simulink model "simulink_a1"  (R2020a)
settings: Solver=FixedStepAuto  StartTime=0.0  StopTime=10.0  FixedStep=1e-3  RelTol=1e-3  EnableMultiTasking=on
undefined symbols (not defined in the file): D0, D1, D10, D11, D12, D13, D2, D3, D4, D5, D6, D7, D8, D9, PTA0, PTA1, PTA2, PTB23, PTB9, PTC16, PTC17, PTC2, PTC3, PTC4, PTD0, PTD1, PTD2, PTD3
libraries: frdmk64flib x18
settings Model: ExtModeTrigDuration=5  Creator=eotte  LastModifiedBy=eotte
settings OptimizationCC: EnhancedBackFolding=on  PassReuseOutputArgsAs=Individual arguments  ZeroExternalMemoryAtStartup=off  ZeroInternalMemoryAtStartup=off  MaxStackSize=64  OptimizeBlockOrder=speed  DifferentSizesBufferReuse=on  OptimizationCustomize=off  EfficientTunableParamExpr=on
settings DebuggingCC: ParameterTunabilityLossMsg=error
settings HardwareCC: ProdBitPerPointer=32  ProdBitPerSizeT=32  ProdBitPerPtrDiffT=32  ProdLargestAtomicInteger=Long  ProdLargestAtomicFloat=Double  ProdWordSize=32  ProdHWDeviceType=ARM Compatible->ARM Cortex
settings SFSimCC: MATLABDynamicMemAlloc=off
settings RTWCC: SystemTargetFile=ert.tlc  HardwareBoard=NXP FRDM-K64F  TemplateMakefile=ert_default_tmf  Toolchain=GNU Tools for ARM Embedded Processors
settings CodeAppCC: ForceParamTrailComments=on  IgnoreCustomStorageClasses=off  OperatorAnnotations=on  SimulinkDataObjDesc=on  SFDataObjDesc=on  InsertBlockDesc=on

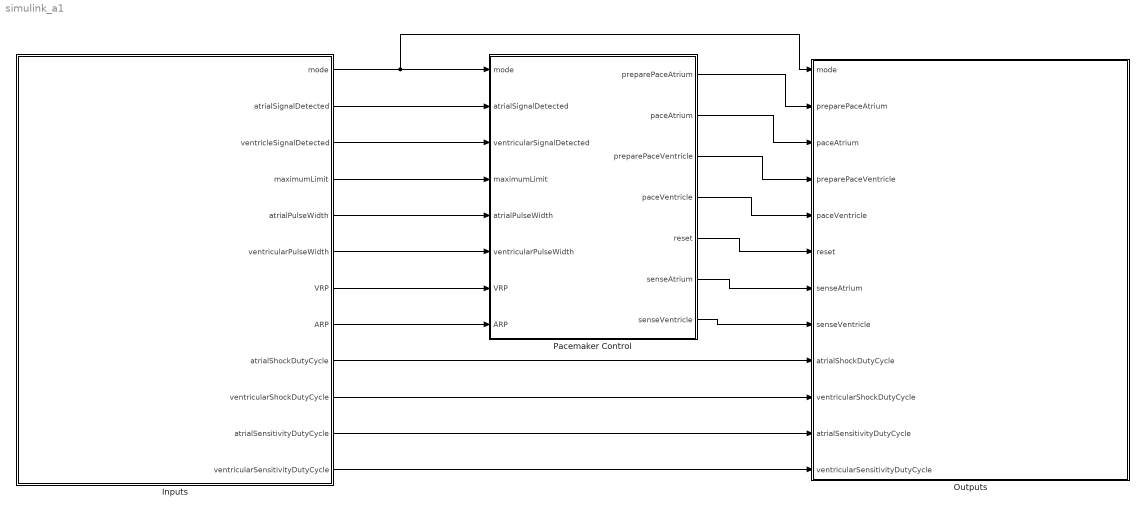
== system simulink_a1 ==
  Inputs : Subsystem
  Outputs : Subsystem
  Pacemaker Control : Stateflow chart  TreatAsAtomicUnit=on
  wires:
  Pacemaker Control/1(preparePaceAtrium) -> Outputs/2(preparePaceAtrium)
  Pacemaker Control/3(preparePaceVentricle) -> Outputs/4(preparePaceVentricle)
  Pacemaker Control/2(paceAtrium) -> Outputs/3(paceAtrium)
  Pacemaker Control/4(paceVentricle) -> Outputs/5(paceVentricle)
  Inputs/1(mode) -> Pacemaker Control/1(mode), Outputs/1(mode)
  Pacemaker Control/5(reset) -> Outputs/6(reset)
  Inputs/2(atrialSignalDetected) -> Pacemaker Control/2(atrialSignalDetected)
  Inputs/3(ventricleSignalDetected) -> Pacemaker Control/3(ventricularSignalDetected)
  Inputs/12(ventricularSensitivityDutyCycle) -> Outputs/12(ventricularSensitivityDutyCycle)
  Inputs/11(atrialSensitivityDutyCycle) -> Outputs/11(atrialSensitivityDutyCycle)
  Inputs/10(ventricularShockDutyCycle) -> Outputs/10(ventricularShockDutyCycle)
  Inputs/9(atrialShockDutyCycle) -> Outputs/9(atrialShockDutyCycle)
  Inputs/4(maximumLimit) -> Pacemaker Control/4(maximumLimit)
  Inputs/5(atrialPulseWidth) -> Pacemaker Control/5(atrialPulseWidth)
  Inputs/6(ventricularPulseWidth) -> Pacemaker Control/6(ventricularPulseWidth)
  Inputs/7(VRP) -> Pacemaker Control/7(VRP)
  Inputs/8(ARP) -> Pacemaker Control/8(ARP)
  Pacemaker Control/6(senseAtrium) -> Outputs/7(senseAtrium)
  Pacemaker Control/7(senseVentricle) -> Outputs/8(senseVentricle)

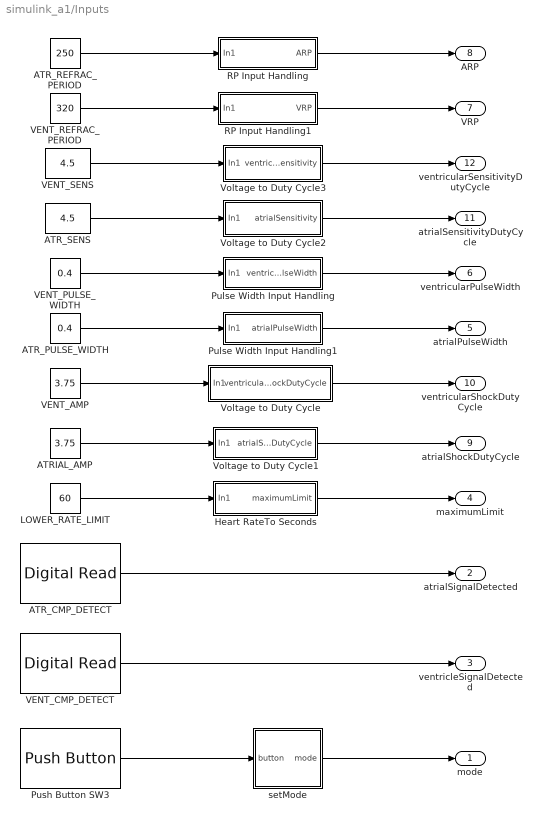
== system simulink_a1/Inputs ==
  ATRIAL_AMP : Constant  Value=3.75
  ATR_CMP_DETECT : frdmk64flib/Digital Read  Whichpin=PTC16 (D0)  SampleTime=-1
  ATR_PULSE_WIDTH : Constant  Value=0.4
  ATR_REFRAC_PERIOD : Constant  Value=250
  ATR_SENS : Constant  Value=4.5
  Heart RateTo Seconds : Subsystem
  LOWER_RATE_LIMIT : Constant  Value=60
  Pulse Width Input Handling : Subsystem
  Pulse Width Input Handling1 : Subsystem
  Push Button SW3 : frdmk64flib/Push Button  Whichswitch=SW3  SampleTime1=-1
  RP Input Handling : Subsystem
  RP Input Handling1 : Subsystem
  VENT_AMP : Constant  Value=3.75
  VENT_CMP_DETECT : frdmk64flib/Digital Read  Whichpin=PTC17 (D1)  SampleTime=-1
  VENT_PULSE_WIDTH : Constant  Value=0.4
  VENT_REFRAC_PERIOD : Constant  Value=320
  VENT_SENS : Constant  Value=4.5
  Voltage to Duty Cycle : Subsystem
  Voltage to Duty Cycle1 : Subsystem
  Voltage to Duty Cycle2 : Subsystem
  Voltage to Duty Cycle3 : Subsystem
  setMode : Stateflow chart  TreatAsAtomicUnit=on
  mode : Outport
  atrialSignalDetected : Outport  Port=2
  ventricleSignalDetected : Outport  Port=3
  maximumLimit : Outport  Port=4
  atrialPulseWidth : Outport  Port=5
  ventricularPulseWidth : Outport  Port=6
  VRP : Outport  Port=7
  ARP : Outport  Port=8
  atrialShockDutyCycle : Outport  Port=9
  ventricularShockDutyCycle : Outport  Port=10
  atrialSensitivityDutyCycle : Outport  Port=11
  ventricularSensitivityDutyCycle : Outport  Port=12
  wires:
  setMode/1(mode) -> mode/1
  Push Button SW3/1 -> setMode/1(button)
  ATR_CMP_DETECT/1 -> atrialSignalDetected/1
  VENT_CMP_DETECT/1 -> ventricleSignalDetected/1
  ATRIAL_AMP/1 -> Voltage to Duty Cycle1/1(In1)
  VENT_AMP/1 -> Voltage to Duty Cycle/1(In1)
  VENT_SENS/1 -> Voltage to Duty Cycle3/1(In1)
  ATR_SENS/1 -> Voltage to Duty Cycle2/1(In1)
  VENT_PULSE_WIDTH/1 -> Pulse Width Input Handling/1(In1)
  LOWER_RATE_LIMIT/1 -> Heart RateTo Seconds/1(In1)
  Heart RateTo Seconds/1(maximumLimit) -> maximumLimit/1
  Voltage to Duty Cycle/1(ventricularShockDutyCycle) -> ventricularShockDutyCycle/1
  Voltage to Duty Cycle1/1(atrialShockDutyCycle) -> atrialShockDutyCycle/1
  Voltage to Duty Cycle3/1(ventricularSensitivity) -> ventricularSensitivityDutyCycle/1
  Voltage to Duty Cycle2/1(atrialSensitivity) -> atrialSensitivityDutyCycle/1
  Pulse Width Input Handling/1(ventricularPulseWidth) -> ventricularPulseWidth/1
  Pulse Width Input Handling1/1(atrialPulseWidth) -> atrialPulseWidth/1
  ATR_PULSE_WIDTH/1 -> Pulse Width Input Handling1/1(In1)
  RP Input Handling1/1(VRP) -> VRP/1
  RP Input Handling/1(ARP) -> ARP/1
  ATR_REFRAC_PERIOD/1 -> RP Input Handling/1(In1)
  VENT_REFRAC_PERIOD/1 -> RP Input Handling1/1(In1)

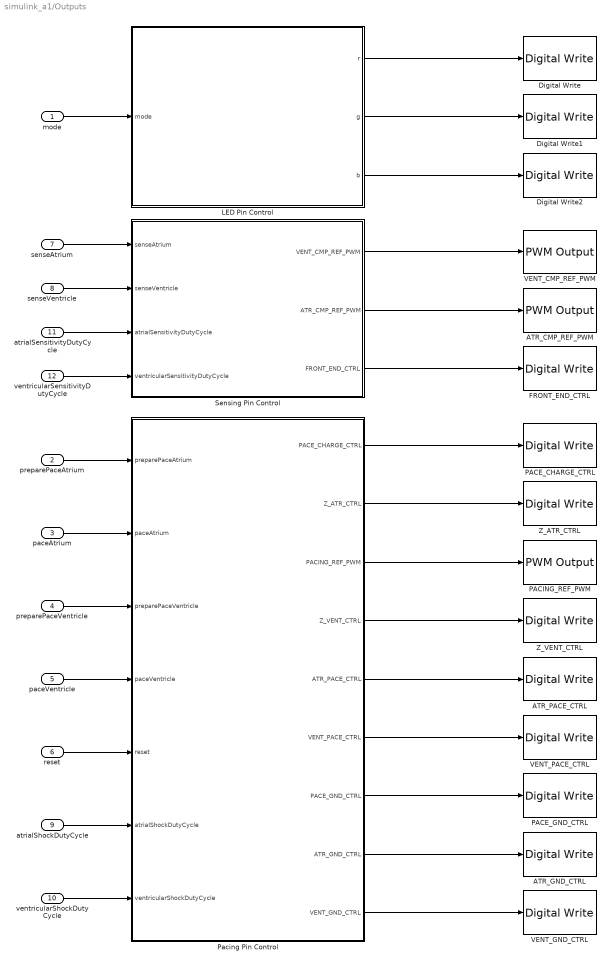
== system simulink_a1/Outputs ==
  mode : Inport
  preparePaceAtrium : Inport  Port=2
  paceAtrium : Inport  Port=3
  preparePaceVentricle : Inport  Port=4
  paceVentricle : Inport  Port=5
  reset : Inport  Port=6
  senseAtrium : Inport  Port=7
  senseVentricle : Inport  Port=8
  atrialShockDutyCycle : Inport  Port=9
  ventricularShockDutyCycle : Inport  Port=10
  atrialSensitivityDutyCycle : Inport  Port=11
  ventricularSensitivityDutyCycle : Inport  Port=12
  ATR_CMP_REF_PWM : frdmk64flib/PWM Output  Whichpin=PTC2 (D6)  InitialFrequency=2000  InitialDutyCycle=0
  ATR_GND_CTRL : frdmk64flib/Digital Write  Whichpin=PTD2 (D11)
  ATR_PACE_CTRL : frdmk64flib/Digital Write  Whichpin=PTA0 (D8)
  Digital Write : frdmk64flib/Digital Write  Whichpin=RED_LED
  Digital Write1 : frdmk64flib/Digital Write  Whichpin=GREEN_LED
  Digital Write2 : frdmk64flib/Digital Write  Whichpin=BLUE_LED
  FRONT_END_CTRL : frdmk64flib/Digital Write  Whichpin=PTD1 (D13)
  LED Pin Control : Stateflow chart  TreatAsAtomicUnit=on
  PACE_CHARGE_CTRL : frdmk64flib/Digital Write  Whichpin=PTB9 (D2)
  PACE_GND_CTRL : frdmk64flib/Digital Write  Whichpin=PTD0 (D10)
  PACING_REF_PWM : frdmk64flib/PWM Output  Whichpin=PTA2 (D5)  InitialFrequency=2000  InitialDutyCycle=0
  Pacing Pin Control : Stateflow chart  TreatAsAtomicUnit=on
      settings: PortSchema="{\"entries\":[{\"content\":{\"sides\":[{\"content\":{\"connectorIds\":[\"In1\",\"In2\",\"In3\",\"In4\",\"In5\",\"In6\",\"In7\"]},\"type\":\"ConnectorPlacement.EquallySpacedRectSide\",\"uuid\":\"92253962-87e9-4e7c-bcdb-24e58fe0c055\"},{\"content\":{\"connectorIds\":[\"Out2\",\"Out8\",\"Out5\",\"Out9\",\"Out3\",\"Out7\",\"Out4\",\"Out1\",\"Out6\"],\"side\":\"RIGHT\"},\"type\":\"ConnectorPlacement.EquallySpacedRectSide\",\"uuid\":\"4cb9541d-32ff-4bb4-8e4b-d9f1d7e76c76\"},{\"content\":{\"connectorIds\":[],\"side\":\"TOP\"},\"type\":\"ConnectorPlacement.EquallySpacedRectSide\",\"uuid\":\"cc690cb9-25b8-4ee8-ae3f-a22909f5e3a8\"},{\"content\":{\"connectorIds\":[],\"side\":\"BOTTOM\"},\"type\":\"ConnectorPlacement.EquallySpacedRectSide\",\"uuid\":\"0aa6c860-c953-4b2e-baf5-040a508b9d07\"}]},\"type\":\"ConnectorPlacement.EquallySpacedConnector\",\"uuid\":\"d7c6b2d5-ade3-439b-b1ea-d68e76d328ac\"}],\"packageUris\":[\"http://schema.mathworks.com/mf0/Connector/19700101\"],\"version\":\"1.0\"}"
  Sensing Pin Control : Stateflow chart  TreatAsAtomicUnit=on
      settings: PortSchema="{\"entries\":[{\"content\":{\"sides\":[{\"content\":{\"connectorIds\":[\"In1\",\"In2\",\"In3\",\"In4\"]},\"type\":\"ConnectorPlacement.EquallySpacedRectSide\",\"uuid\":\"f0f6a072-4109-4fa4-bc82-6d6350130513\"},{\"content\":{\"connectorIds\":[\"Out3\",\"Out2\",\"Out1\"],\"side\":\"RIGHT\"},\"type\":\"ConnectorPlacement.EquallySpacedRectSide\",\"uuid\":\"04a191da-9ef7-404f-bbc7-e2275fa0f798\"},{\"content\":{\"connectorIds\":[],\"side\":\"TOP\"},\"type\":\"ConnectorPlacement.EquallySpacedRectSide\",\"uuid\":\"3258143e-ec04-4818-a8fd-7397dd93120a\"}]},\"type\":\"ConnectorPlacement.EquallySpacedConnector\",\"uuid\":\"abd9187b-7230-471c-b20b-6fa4748c984d\"}],\"packageUris\":[\"http://schema.mathworks.com/mf0/Connector/19700101\"],\"version\":\"1.0\"}"
  VENT_CMP_REF_PWM : frdmk64flib/PWM Output  Whichpin=PTA1 (D3)  InitialFrequency=2000  InitialDutyCycle=0
  VENT_GND_CTRL : frdmk64flib/Digital Write  Whichpin=PTD3 (D12)
  VENT_PACE_CTRL : frdmk64flib/Digital Write  Whichpin=PTC4 (D9)
  Z_ATR_CTRL : frdmk64flib/Digital Write  Whichpin=PTB23 (D4)
  Z_VENT_CTRL : frdmk64flib/Digital Write  Whichpin=PTC3 (D7)
  wires:
  preparePaceAtrium/1 -> Pacing Pin Control/1(preparePaceAtrium)
  paceAtrium/1 -> Pacing Pin Control/2(paceAtrium)
  preparePaceVentricle/1 -> Pacing Pin Control/3(preparePaceVentricle)
  paceVentricle/1 -> Pacing Pin Control/4(paceVentricle)
  Pacing Pin Control/1(ATR_GND_CTRL) -> ATR_GND_CTRL/1
  Pacing Pin Control/2(PACE_CHARGE_CTRL) -> PACE_CHARGE_CTRL/1
  Pacing Pin Control/3(ATR_PACE_CTRL) -> ATR_PACE_CTRL/1
  Pacing Pin Control/5(PACING_REF_PWM) -> PACING_REF_PWM/1
  Pacing Pin Control/8(Z_ATR_CTRL) -> Z_ATR_CTRL/1
  Pacing Pin Control/4(PACE_GND_CTRL) -> PACE_GND_CTRL/1
  Pacing Pin Control/6(VENT_GND_CTRL) -> VENT_GND_CTRL/1
  Pacing Pin Control/9(Z_VENT_CTRL) -> Z_VENT_CTRL/1
  Pacing Pin Control/7(VENT_PACE_CTRL) -> VENT_PACE_CTRL/1
  reset/1 -> Pacing Pin Control/5(reset)
  atrialShockDutyCycle/1 -> Pacing Pin Control/6(atrialShockDutyCycle)
  ventricularShockDutyCycle/1 -> Pacing Pin Control/7(ventricularShockDutyCycle)
  LED Pin Control/2(g) -> Digital Write1/1
  LED Pin Control/1(r) -> Digital Write/1
  LED Pin Control/3(b) -> Digital Write2/1
  mode/1 -> LED Pin Control/1(mode)
  senseVentricle/1 -> Sensing Pin Control/2(senseVentricle)
  senseAtrium/1 -> Sensing Pin Control/1(senseAtrium)
  atrialSensitivityDutyCycle/1 -> Sensing Pin Control/3(atrialSensitivityDutyCycle)
  ventricularSensitivityDutyCycle/1 -> Sensing Pin Control/4(ventricularSensitivityDutyCycle)
  Sensing Pin Control/1(FRONT_END_CTRL) -> FRONT_END_CTRL/1
  Sensing Pin Control/2(ATR_CMP_REF_PWM) -> ATR_CMP_REF_PWM/1
  Sensing Pin Control/3(VENT_CMP_REF_PWM) -> VENT_CMP_REF_PWM/1

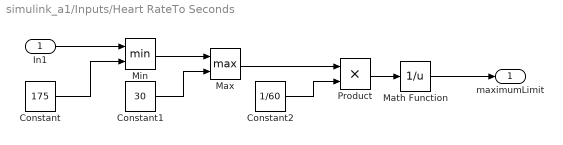
== system simulink_a1/Inputs/Heart RateTo Seconds ==
  In1 : Inport
  Constant : Constant  Value=175
  Constant1 : Constant  Value=30
  Constant2 : Constant  Value=1/60
  Math Function : Math  Operator=reciprocal  SaturateOnIntegerOverflow=on
  Max : MinMax  Function=max  Inputs=2
  Min : MinMax  Inputs=2
  Product : Product
  maximumLimit : Outport
  wires:
  Product/1 -> Math Function/1
  Constant2/1 -> Product/2
  Math Function/1 -> maximumLimit/1
  In1/1 -> Min/1
  Min/1 -> Max/1
  Max/1 -> Product/1
  Constant/1 -> Min/2
  Constant1/1 -> Max/2

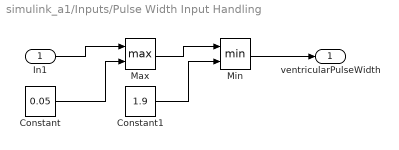
== system simulink_a1/Inputs/Pulse Width Input Handling ==
  In1 : Inport
  Constant : Constant  Value=0.05
  Constant1 : Constant  Value=1.9
  Max : MinMax  Function=max  Inputs=2
  Min : MinMax  Inputs=2
  ventricularPulseWidth : Outport
  wires:
  Max/1 -> Min/1
  In1/1 -> Max/1
  Min/1 -> ventricularPulseWidth/1
  Constant/1 -> Max/2
  Constant1/1 -> Min/2

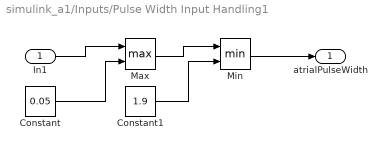
== system simulink_a1/Inputs/Pulse Width Input Handling1 ==
  In1 : Inport
  Constant : Constant  Value=0.05
  Constant1 : Constant  Value=1.9
  Max : MinMax  Function=max  Inputs=2
  Min : MinMax  Inputs=2
  atrialPulseWidth : Outport
  wires:
  Max/1 -> Min/1
  In1/1 -> Max/1
  Min/1 -> atrialPulseWidth/1
  Constant/1 -> Max/2
  Constant1/1 -> Min/2

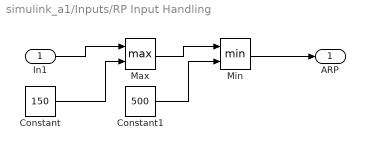
== system simulink_a1/Inputs/RP Input Handling ==
  In1 : Inport
  Constant : Constant  Value=150
  Constant1 : Constant  Value=500
  Max : MinMax  Function=max  Inputs=2
  Min : MinMax  Inputs=2
  ARP : Outport
  wires:
  Max/1 -> Min/1
  In1/1 -> Max/1
  Min/1 -> ARP/1
  Constant/1 -> Max/2
  Constant1/1 -> Min/2

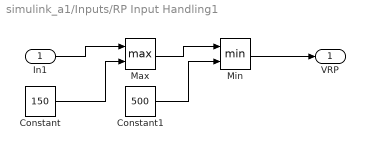
== system simulink_a1/Inputs/RP Input Handling1 ==
  In1 : Inport
  Constant : Constant  Value=150
  Constant1 : Constant  Value=500
  Max : MinMax  Function=max  Inputs=2
  Min : MinMax  Inputs=2
  VRP : Outport
  wires:
  Max/1 -> Min/1
  In1/1 -> Max/1
  Min/1 -> VRP/1
  Constant/1 -> Max/2
  Constant1/1 -> Min/2

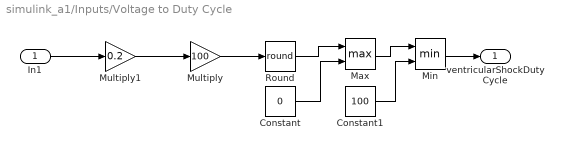
== system simulink_a1/Inputs/Voltage to Duty Cycle ==
  In1 : Inport
  Constant : Constant  Value=0
  Constant1 : Constant  Value=100
  Max : MinMax  Function=max  Inputs=2
  Min : MinMax  Inputs=2
  Multiply : Gain  Gain=100
  Multiply1 : Gain  Gain=0.2
  Round : Rounding  Operator=round
  ventricularShockDutyCycle : Outport
  wires:
  In1/1 -> Multiply1/1
  Multiply1/1 -> Multiply/1
  Multiply/1 -> Round/1
  Round/1 -> Max/1
  Max/1 -> Min/1
  Min/1 -> ventricularShockDutyCycle/1
  Constant/1 -> Max/2
  Constant1/1 -> Min/2

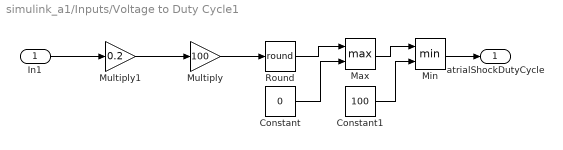
== system simulink_a1/Inputs/Voltage to Duty Cycle1 ==
  In1 : Inport
  Constant : Constant  Value=0
  Constant1 : Constant  Value=100
  Max : MinMax  Function=max  Inputs=2
  Min : MinMax  Inputs=2
  Multiply : Gain  Gain=100
  Multiply1 : Gain  Gain=0.2
  Round : Rounding  Operator=round
  atrialShockDutyCycle : Outport
  wires:
  In1/1 -> Multiply1/1
  Multiply1/1 -> Multiply/1
  Multiply/1 -> Round/1
  Round/1 -> Max/1
  Max/1 -> Min/1
  Min/1 -> atrialShockDutyCycle/1
  Constant/1 -> Max/2
  Constant1/1 -> Min/2

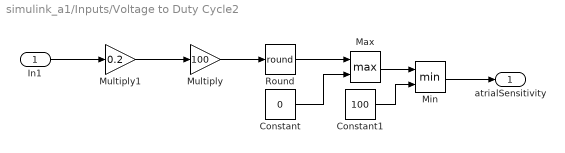
== system simulink_a1/Inputs/Voltage to Duty Cycle2 ==
  In1 : Inport
  Constant : Constant  Value=0
  Constant1 : Constant  Value=100
  Max : MinMax  Function=max  Inputs=2
  Min : MinMax  Inputs=2
  Multiply : Gain  Gain=100
  Multiply1 : Gain  Gain=0.2
  Round : Rounding  Operator=round
  atrialSensitivity : Outport
  wires:
  In1/1 -> Multiply1/1
  Multiply1/1 -> Multiply/1
  Multiply/1 -> Round/1
  Round/1 -> Max/1
  Max/1 -> Min/1
  Min/1 -> atrialSensitivity/1
  Constant/1 -> Max/2
  Constant1/1 -> Min/2

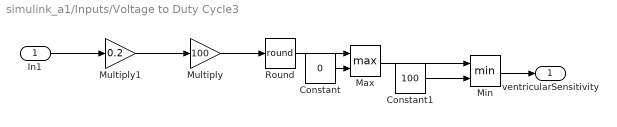
== system simulink_a1/Inputs/Voltage to Duty Cycle3 ==
  In1 : Inport
  Constant : Constant  Value=0
  Constant1 : Constant  Value=100
  Max : MinMax  Function=max  Inputs=2
  Min : MinMax  Inputs=2
  Multiply : Gain  Gain=100
  Multiply1 : Gain  Gain=0.2
  Round : Rounding  Operator=round
  ventricularSensitivity : Outport
  wires:
  In1/1 -> Multiply1/1
  Multiply1/1 -> Multiply/1
  Multiply/1 -> Round/1
  Round/1 -> Max/1
  Max/1 -> Min/1
  Min/1 -> ventricularSensitivity/1
  Constant/1 -> Max/2
  Constant1/1 -> Min/2

== stateflow chart simulink_a1/Inputs/setMode ==
  state AOO
    entry:
    mode = 100;
  state Off
    entry:
    mode = 0;
  state VOO
    entry:
    mode = 200;
  state VVI
    entry:
    mode = 221;
  state AAI
    entry:
    mode = 111;
  (default) -> Off
  Off -> AOO : [button == 1 && after(1,sec)]
  VVI -> Off : [button == 1 && after(1,sec)]
  AOO -> VOO : [button == 1 && after(1,sec)]
  AAI -> VVI : [button == 1 && after(1,sec)]
  VOO -> AAI : [button == 1 && after(1,sec)]
  data: mode output; button input

== stateflow chart simulink_a1/Pacemaker Control ==
  state AOO
    state Shock
      entry:
      paceAtrium = true;
      exit:
      paceAtrium = false;
    state Prep
      entry:
      preparePaceAtrium = true;
      exit:
      preparePaceAtrium = false;
    (default) -> AOO.Prep
    AOO.Prep -> AOO.Shock : [after(maximumLimit,sec)]
    AOO.Shock -> AOO.Prep : [after(atrialPulseWidth,msec)]
  state VOO
    state Shock
      entry:
      paceVentricle = true;
      exit:
      paceVentricle = false;
    state Prep
      entry:
      preparePaceVentricle = true;
      exit:
      preparePaceVentricle = false;
    (default) -> VOO.Prep
    VOO.Prep -> VOO.Shock : [after(maximumLimit,sec)]
    VOO.Shock -> VOO.Prep : [after(ventricularPulseWidth,msec)]
  state Off
    entry:
    reset = true;
    preparePaceAtrium = false;
    paceAtrium = false;
    preparePaceVentricle = false;
    paceVentricle = false;
    senseAtrium = false;
    senseVentricle = false;
    exit:
    reset = false;
  state AAI
    state Pace
      entry:
      paceAtrium = true;
      exit:
      paceAtrium = false;
    state Sense
      entry:
      preparePaceAtrium = true;
      senseAtrium = true;
      exit:
      preparePaceAtrium = false;
    (default) -> AAI.Sense
    AAI.Sense -> AAI.Sense [order 2] : [atrialSignalDetected && after(ARP, msec)]
    AAI.Sense -> AAI.Pace [order 1] : [after(maximumLimit, sec) && after(ARP, msec)]
    AAI.Pace -> AAI.Sense : [after(atrialPulseWidth,msec)]
  state VVI
    state Pace
      entry:
      paceVentricle = true;
      exit:
      paceVentricle = false;
    state Sense
      entry:
      preparePaceVentricle = true;
      senseVentricle = true;
      exit:
      preparePaceVentricle = false;
    (default) -> VVI.Sense
    VVI.Sense -> VVI.Sense [order 2] : [ventricularSignalDetected && after(VRP, msec)]
    VVI.Sense -> VVI.Pace [order 1] : [after(maximumLimit, sec) && after(VRP, msec)]
    VVI.Pace -> VVI.Sense : [after(ventricularPulseWidth, msec)]
  AOO -> Off : [mode ~= 100]
  Off -> AOO [order 3] : [mode ==100]
  Off -> VOO [order 4] : [mode == 200]
  VOO -> Off : [mode ~= 200]
  (default) -> Off
  AAI -> Off : [mode ~= 111]
  Off -> AAI [order 1] : [mode == 111]
  VVI -> Off : [mode ~= 221]
  Off -> VVI [order 2] : [mode == 221]
  data: preparePaceAtrium output; paceAtrium output; preparePaceVentricle output; paceVentricle output; mode input; reset output; atrialSignalDetected input; ventricularSignalDetected input; maximumLimit input; atrialPulseWidth input; ventricularPulseWidth input; VRP input; ARP input; senseAtrium output; senseVentricle output

== stateflow chart simulink_a1/Outputs/LED Pin Control ==
  state AOO
    entry:
    r = true;
    g = false;
    b = false;
  state Off
    entry:
    r = true;
    g = true;
    b = true;
  state VOO
    entry:
    r = false;
    g = true;
    b = false;
  state VVI
    entry:
    r = false;
    g = false;
    b = true;
  state AAI
    entry:
    r = true;
    g = false;
    b = true;
  (default) -> Off
  Off -> AOO : [mode ~= 0]
  VVI -> Off : [mode ~= 221]
  AOO -> VOO : [mode ~= 100]
  AAI -> VVI : [mode ~= 111]
  VOO -> AAI : [mode ~= 200]
  data: mode input; r output; g output; b output

== stateflow chart simulink_a1/Outputs/Sensing Pin Control ==
  state SenseAtrium
    entry:
    VENT_CMP_REF_PWM = 0;
    ATR_CMP_REF_PWM = atrialSensitivityDutyCycle;
    FRONT_END_CTRL = true;
  state Default
    entry:
    %Set all pins to 0/false
    FRONT_END_CTRL = true;
    VENT_CMP_REF_PWM = 0;
    ATR_CMP_REF_PWM = 0;
  state SenseVentricle
    entry:
    ATR_CMP_REF_PWM = 0;
    VENT_CMP_REF_PWM = ventricularSensitivityDutyCycle;
    FRONT_END_CTRL = true;
  Default -> SenseAtrium [order 1] : [senseAtrium]
  SenseAtrium -> Default : [~senseAtrium]
  (default) -> Default
  Default -> SenseVentricle [order 2] : [senseVentricle]
  SenseVentricle -> Default : [~senseVentricle]
  data: FRONT_END_CTRL output; senseAtrium input; senseVentricle input; atrialSensitivityDutyCycle input; ventricularSensitivityDutyCycle input; ATR_CMP_REF_PWM output; VENT_CMP_REF_PWM output

== stateflow chart simulink_a1/Outputs/Pacing Pin Control ==
  state PreparePaceAtrium
    entry:
    %Charging C22
    VENT_PACE_CTRL = false;
    ATR_PACE_CTRL = false;
    PACING_REF_PWM = atrialShockDutyCycle;
    PACE_CHARGE_CTRL = true;
    %Discharging C21
    PACE_GND_CTRL = true;
    Z_VENT_CTRL = false;
    Z_ATR_CTRL = false;
    ATR_GND_CTRL = true;
    %All other pins
    VENT_GND_CTRL = false;
  state Default
    entry:
    %Set all pins to 0 or false
    VENT_PACE_CTRL = false;
    ATR_PACE_CTRL = false;
    PACING_REF_PWM = 0;
    PACE_CHARGE_CTRL = false;
    PACE_GND_CTRL = false;
    Z_VENT_CTRL = false;
    Z_ATR_CTRL = false;
    ATR_GND_CTRL = false;
    VENT_GND_CTRL = false;
  state PreparePaceVentricle
    entry:
    %Charging C22
    ATR_PACE_CTRL = false;
    VENT_PACE_CTRL = false;
    PACING_REF_PWM = ventricularShockDutyCycle;
    PACE_CHARGE_CTRL = true;
    %Discharging C21
    PACE_GND_CTRL = true;
    Z_ATR_CTRL = false;
    Z_VENT_CTRL = false;
    VENT_GND_CTRL = true;
    %All other pins
    ATR_GND_CTRL = false;
  state PaceVentricle
    entry:
    %Discharging C22
    PACE_CHARGE_CTRL = false;
    PACE_GND_CTRL = true;
    ATR_PACE_CTRL = false;
    ATR_GND_CTRL = false;
    Z_ATR_CTRL = false;
    Z_VENT_CTRL = false;
    VENT_GND_CTRL = false;
    VENT_PACE_CTRL = true;
    %All other pins
    PACING_REF_PWM = 0;
  state PaceAtrium
    entry:
    %Discharging C22
    PACE_CHARGE_CTRL = false;
    PACE_GND_CTRL = true;
    VENT_PACE_CTRL = false;
    VENT_GND_CTRL = false;
    Z_VENT_CTRL = false;
    Z_ATR_CTRL = false;
    ATR_GND_CTRL = false;
    ATR_PACE_CTRL = true;
    %All other pins
    PACING_REF_PWM = 0;
  (default) -> Default
  Default -> PreparePaceVentricle [order 2] : [preparePaceVentricle]
  Default -> PreparePaceAtrium [order 1] : [preparePaceAtrium]
  PreparePaceVentricle -> Default [order 2] : [reset == true]
  PreparePaceAtrium -> Default [order 2] : [reset == true]
  PaceVentricle -> PreparePaceVentricle [order 1] : [preparePaceVentricle]
  PreparePaceVentricle -> PaceVentricle [order 1] : [paceVentricle]
  PaceAtrium -> Default [order 2] : [reset== true]
  PaceVentricle -> Default [order 2] : [reset == true]
  PaceAtrium -> PreparePaceAtrium [order 1] : [preparePaceAtrium]
  PreparePaceAtrium -> PaceAtrium [order 1] : [paceAtrium]
  data: preparePaceAtrium input; paceAtrium input; preparePaceVentricle input; paceVentricle input; ATR_GND_CTRL output; PACE_CHARGE_CTRL output; ATR_PACE_CTRL output; PACE_GND_CTRL output; PACING_REF_PWM output; VENT_GND_CTRL output; VENT_PACE_CTRL output; Z_ATR_CTRL output; Z_VENT_CTRL output; reset input; atrialShockDutyCycle input; ventricularShockDutyCycle input
